simulink model "model"  (R2021a)
settings: Solver=VariableStepAuto  StartTime=0.0  StopTime=100  RelTol=1e-3
values from neighbouring files (symbols this model uses):
  C = eye(12)    [init.m]
  I = [Jx Jxy Jxz ... (first row only)    [init.m]
  m = 1.5    [init.m]
undefined symbols (not defined in the file or in its folder): DiscIntNeverNeededParam, K_lqr, PID_pitch, PID_roll, PID_yaw
libraries: simulink x3
settings Model: Creator=iris  LastModifiedBy=iris

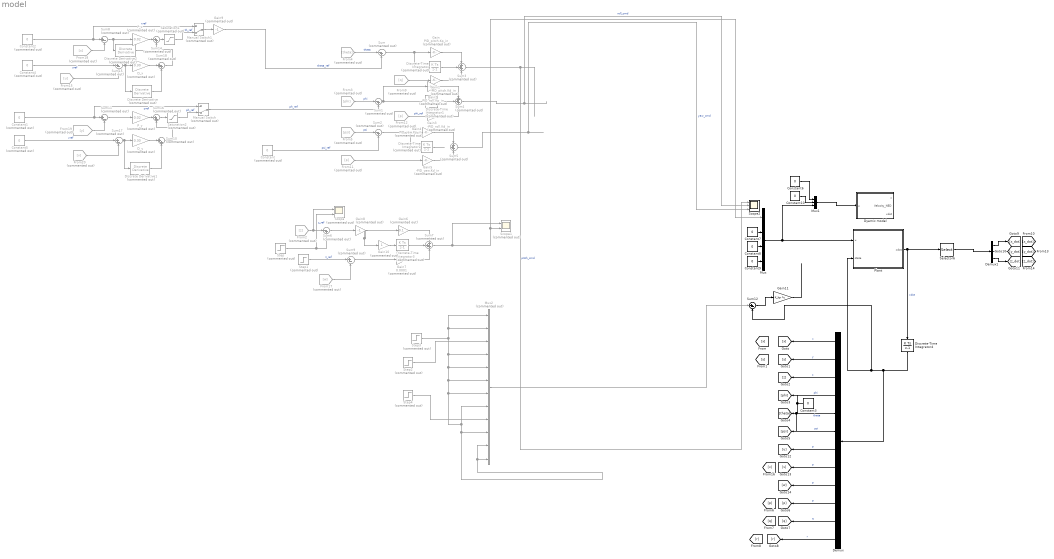
== system model ==
  Constant{,1..2,4..5} (5 alike) : Constant  Commented=on  Value=0
  Constant{3,6..10} (6 alike) : Constant  Value=0
  D_x : Gain  Commented=on  Gain=0.30
  D_y : Gain  Commented=on  Gain=0.30
  Demux : Demux  Outputs=12
  Demux1 : Demux  Outputs=3
  Discrete Derivative : simulink/Discrete/Discrete Derivative  Commented=on  gainval=0.1  ICPrevScaledInput=0.0  OutMin=[]  OutMax=[]  OutDataType=fixdt(1, 16)  OutScaling=2^-10  DoSatur=off
  Discrete Derivative1 : simulink/Discrete/Discrete Derivative  Commented=on  gainval=0.1  ICPrevScaledInput=0.0  OutMin=[]  OutMax=[]  OutDataType=fixdt(1, 16)  OutScaling=2^-10  DoSatur=off
  Discrete Derivative2 : simulink/Discrete/Discrete Derivative  Commented=on  gainval=0.08  ICPrevScaledInput=0.0  OutMin=[]  OutMax=[]  OutDataType=fixdt(1, 16)  OutScaling=2^-10  DoSatur=off
  Discrete-Time Integrator : DiscreteIntegrator  Commented=on  gainval=PID_pitch.Ki_in  SampleTime=-1  ICPrevOutput=DiscIntNeverNeededParam  ICPrevScaledInput=DiscIntNeverNeededParam
  Discrete-Time Integrator1 : DiscreteIntegrator  Commented=on  gainval=PID_roll.Ki_in  SampleTime=-1  ICPrevOutput=DiscIntNeverNeededParam  ICPrevScaledInput=DiscIntNeverNeededParam
  Discrete-Time Integrator2 : DiscreteIntegrator  Commented=on  gainval=PID_yaw.Ki_in  SampleTime=-1  UpperSaturationLimit=0.2  LowerSaturationLimit=-0.2  ICPrevOutput=DiscIntNeverNeededParam  ICPrevScaledInput=DiscIntNeverNeededParam
  Discrete-Time Integrator3 : DiscreteIntegrator  Commented=on  gainval=0.001  SampleTime=-1  ICPrevOutput=DiscIntNeverNeededParam  ICPrevScaledInput=DiscIntNeverNeededParam
  Discrete-Time Integrator4 : DiscreteIntegrator  SampleTime=-1  ICPrevOutput=DiscIntNeverNeededParam  ICPrevScaledInput=DiscIntNeverNeededParam
  Dyamic model : Subsystem
  From11 : From  Commented=on  GotoTag=p
  From12 : From  Commented=on  GotoTag=p
  From15 : From  Commented=on  GotoTag=u
  From17 : From  Commented=on  GotoTag=w
  From18 : From  Commented=on  GotoTag=x
  From19 : From  Commented=on  GotoTag=y
  From2 : From  Commented=on  GotoTag=z
  From20 : From  Commented=on  GotoTag=v
  From3 : From  Commented=on  GotoTag=phi
  From4 : From  Commented=on  GotoTag=theta
  From5 : From  Commented=on  GotoTag=psi
  From9 : From  Commented=on  GotoTag=q
  Gain : Gain  Commented=on  Gain=PID_pitch.Kp_in
  Gain1 : Gain  Commented=on  Gain=-PID_pitch.Kd_in
  Gain10 : Gain  Commented=on
  Gain11 : Gain  Gain=K_lqr  Multiplication=Matrix(K*u)
  Gain2 : Gain  Commented=on  Gain=PID_roll.Kp_in
  Gain3 : Gain  Commented=on  Gain=-PID_roll.Kd_in
  Gain4 : Gain  Commented=on  Gain=PID_yaw.Kp_in
  Gain5 : Gain  Commented=on  Gain=-PID_yaw.Kd_in
  Gain6 : Gain  Commented=on  Gain=0.1
  Gain7 : Gain  Commented=on  Gain=0.0001
  Gain8 : Gain  Commented=on  Gain=-1
  Gain9 : Gain  Commented=on  Gain=-1
  Manual Switch : ManualSwitch  Commented=on  CurrentSetting=0
  Manual Switch1 : ManualSwitch  Commented=on  CurrentSetting=0
  Mux : Mux
  Mux1 : Mux  Inputs=3
  Mux2 : Mux  Commented=on  Inputs=12
  P_x : Gain  Commented=on  Gain=0.02
  P_y : Gain  Commented=on  Gain=0.02
  Plant : Subsystem
  Saturation1 : Saturate  Commented=on  UpperLimit=30/180*pi  LowerLimit=-30/180*pi
  Saturation2 : Saturate  Commented=on  UpperLimit=30/180*pi  LowerLimit=-30/180*pi
  Scope : Scope  Commented=on  NumInputPorts=2
  Scope1 : Scope  Commented=on  NumInputPorts=2
  Scope2 : Scope  NumInputPorts=3
  Selector6 : Selector  InputPortWidth=12  IndexOptions=Index vector (dialog)  Indices=[1:3]  OutputSizes=1
  Step : Step  Commented=on  SampleTime=0
  Step1 : Step  Commented=on  After=0.1  SampleTime=0
  Step2 : Step  Commented=on  SampleTime=0
  Step3 : Step  Commented=on  After=0  SampleTime=0
  Step4 : Step  Commented=on  After=0.1  SampleTime=0
  Sum{,1..2,6} (4 alike) : Sum  Commented=on  Inputs=|-+
  Sum{10,14,16,18} (4 alike) : Sum  Commented=on  Inputs=|++
  Sum{8..9,11,15,17} (5 alike) : Sum  Commented=on  Inputs=|+-
  Sum12 : Sum  Inputs=|+-
  Sum{3..5,7} (4 alike) : Sum  Commented=on  Inputs=+++
  wires:
  Mux/1 -> Plant/1(u), Mux1/3
  Plant/1(xdot) -> Discrete-Time Integrator4/1, Selector6/1  "xdot"
  Demux/1 -> [x]  "x"
  Demux/2 -> [y]  "y"
  Demux/12 -> [r]  "r"
  Demux/4 -> ?  "phi"
  Demux/5 -> ?  "theta"
  Demux/6 -> ?  "psi"
  Demux/10 -> [p]  "p"
  Demux/11 -> [q]  "q"
  From3/1 -> Sum1/1  "phi"
  From5/1 -> Sum2/1  "psi"
  From4/1 -> Sum/1  "theta"
  Demux/3 -> [z]  "z"
  Discrete-Time Integrator/1 -> Sum3/2
  From9/1 -> Gain1/1
  Sum/1 -> Discrete-Time Integrator/1, Gain/1
  Gain1/1 -> Sum3/3
  Constant/1 -> Sum2/2  "psi_ref"
  Gain/1 -> Sum3/1
  Gain3/1 -> Sum4/3
  Gain2/1 -> Sum4/1
  Discrete-Time Integrator1/1 -> Sum4/2
  Sum1/1 -> Gain2/1, Discrete-Time Integrator1/1
  From12/1 -> Gain3/1  "phi_ref"
  Gain4/1 -> Sum5/1
  Sum2/1 -> Discrete-Time Integrator2/1, Gain4/1
  Discrete-Time Integrator2/1 -> ?
  From11/1 -> Gain5/1
  Gain5/1 -> Sum5/3
  Sum3/1 -> Scope2/1  "pitch_cmd"
  Sum4/1 -> Scope2/2  "roll_cmd"
  Sum5/1 -> Scope2/3  "yaw_cmd"
  Discrete-Time Integrator3/1 -> Sum7/2
  Gain6/1 -> Sum7/1
  Gain8/1 -> Gain10/1, Gain6/1
  Gain7/1 -> Sum7/3
  Sum6/1 -> Gain8/1
  Selector6/1 -> Demux1/1
  Demux1/1 -> [x_dot]
  Demux1/2 -> [y_dot]
  Demux1/3 -> [z_dot]
  From17/1 -> Sum9/2
  From2/1 -> Scope/1, Sum6/1
  Step/1 -> Scope/2, Sum6/2  "z_ref"
  Gain9/1 -> Sum/2  "theta_ref"
  Demux/7 -> [u]  "p"
  Demux/8 -> [v]  "p"
  Demux/9 -> [w]  "p"
  Manual Switch1/1 -> Gain9/1
  Sum17/1 -> Discrete Derivative1/1, D_y/1
  From18/1 -> Sum8/2
  Saturation2/1 -> Manual Switch/2  "ph_ref"
  Constant4/1 -> Sum15/1  "uref"
  Constant5/1 -> Sum17/1  "vref"
  From20/1 -> Sum17/2
  Sum10/1 -> Sum16/2
  Discrete Derivative/1 -> Sum18/2
  Sum11/1 -> P_y/1
  Discrete Derivative2/1 -> ?
  Sum8/1 -> Discrete Derivative2/1, P_x/1
  P_x/1 -> Sum14/1
  D_y/1 -> Sum10/1
  Discrete Derivative1/1 -> Sum10/2
  Saturation1/1 -> Manual Switch1/2  "th_ref"
  Sum15/1 -> Discrete Derivative/1, D_x/1
  From15/1 -> Sum15/2
  Constant2/1 -> Manual Switch1/1, Sum8/1  "xref"
  Constant1/1 -> Manual Switch/1, Sum11/1  "yref"
  From19/1 -> Sum11/2
  D_x/1 -> Sum18/1
  Sum14/1 -> Saturation1/1
  Manual Switch/1 -> Sum1/2  "ph_ref"
  P_y/1 -> Sum16/1
  Sum16/1 -> Saturation2/1
  Sum18/1 -> Sum14/2
  Constant7/1 -> Mux/2
  Constant8/1 -> Mux/3
  Constant9/1 -> Mux/4
  Sum9/1 -> Gain7/1
  Sum7/1 -> Mux/1, Scope1/2, Scope1/1
  Step1/1 -> Sum9/1  "z_ref"
  Constant3/1 -> [psi], [theta], [phi]
  Constant10/1 -> Mux1/2
  Constant6/1 -> Mux1/1
  Mux1/1 -> Dyamic model/1(u)
  Gain10/1 -> Discrete-Time Integrator3/1
  Mux2/1 -> Sum12/1
  Sum12/1 -> Gain11/1
  Discrete-Time Integrator4/1 -> Demux/1, Sum12/2, Plant/2(state)
  Gain11/1 -> ?
  Step3/1 -> Mux2/2, Mux2/1, Mux2/11, Mux2/12, Mux2/10, Mux2/8, Mux2/7, Mux2/6, Mux2/5, Mux2/4
  Step2/1 -> Mux2/3
  Step4/1 -> Mux2/9

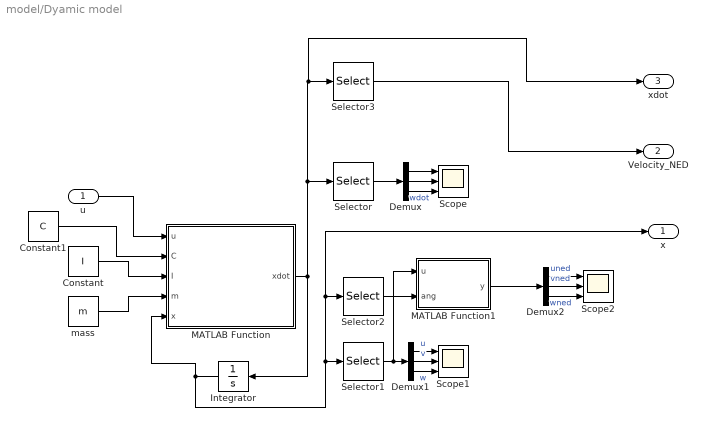
== system model/Dyamic model ==
  u : Inport
  Constant : Constant  Value=I
  Constant1 : Constant  Value=C
  Demux : Demux  Outputs=3
  Demux1 : Demux  Outputs=3
  Demux2 : Demux  Outputs=3
  Integrator : Integrator
  MATLAB Function : MATLAB Function  TreatAsAtomicUnit=on
  MATLAB Function1 : MATLAB Function  TreatAsAtomicUnit=on
  Scope : Scope  NumInputPorts=3
  Scope1 : Scope  NumInputPorts=3
  Scope2 : Scope  NumInputPorts=3
  Selector : Selector  InputPortWidth=12  IndexOptions=Index vector (dialog)  Indices=[7:9]  OutputSizes=1
  Selector1 : Selector  InputPortWidth=12  IndexOptions=Index vector (dialog)  Indices=[7:9]  OutputSizes=1
  Selector2 : Selector  InputPortWidth=12  IndexOptions=Index vector (dialog)  Indices=[4:6]  OutputSizes=1
  Selector3 : Selector  InputPortWidth=12  IndexOptions=Index vector (dialog)  Indices=[1:3]  OutputSizes=1
  mass : Constant  Value=m
  x : Outport  VectorParamsAs1DForOutWhenUnconnected=off
  Velocity_NED : Outport  Port=2  VectorParamsAs1DForOutWhenUnconnected=off
  xdot : Outport  Port=3  VectorParamsAs1DForOutWhenUnconnected=off
  wires:
  mass/1 -> MATLAB Function/4(m)
  MATLAB Function/1(xdot) -> xdot/1, Selector3/1, Selector/1, Integrator/1
  u/1 -> MATLAB Function/1(u)
  Constant/1 -> MATLAB Function/3(I)
  Demux/1 -> Scope/1
  Demux/2 -> Scope/2
  Demux/3 -> Scope/3  "wdot"
  Selector/1 -> Demux/1
  Integrator/1 -> Selector2/1, x/1, Selector1/1, MATLAB Function/5(x)
  Selector1/1 -> MATLAB Function1/1(u), Demux1/1
  Demux1/1 -> Scope1/1  "u"
  Demux1/2 -> Scope1/2  "v"
  Demux1/3 -> Scope1/3  "w"
  Demux2/1 -> Scope2/1  "uned"
  Demux2/2 -> Scope2/2  "vned"
  Demux2/3 -> Scope2/3  "wned"
  MATLAB Function1/1(y) -> Demux2/1
  Selector2/1 -> MATLAB Function1/2(ang)
  Selector3/1 -> Velocity_NED/1
  Constant1/1 -> MATLAB Function/2(C)

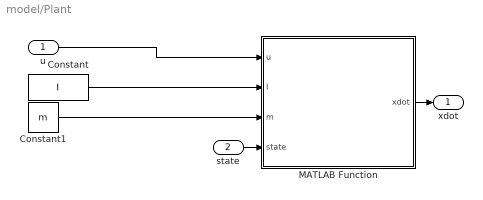
== system model/Plant ==
  u : Inport
  state : Inport  Port=2
  Constant : Constant  Value=I
  Constant1 : Constant  Value=m
  MATLAB Function : MATLAB Function  TreatAsAtomicUnit=on
  xdot : Outport
  wires:
  u/1 -> MATLAB Function/1(u)
  Constant1/1 -> MATLAB Function/3(m)
  MATLAB Function/1(xdot) -> xdot/1
  Constant/1 -> MATLAB Function/2(I)
  state/1 -> MATLAB Function/4(state)

== matlab function model/Dyamic model/MATLAB Function ==
  data: u input; C input; I input; m input; x input; xdot output
function xdot = quadrotor_dynamics(u,C,I,m,x)

ph = x(4);
th = x(5);
ps = x(6);
U = x(7);
V = x(8);
W = x(9);
p = x(10);
q = x(11);
r = x(12);
% Rotation from body to NED
% Rb_ned = [cos(th)*cos(ps), -cos(ph)*sin(ps) + sin(ph)*sin(th)*...
%                 cos(ps), sin(ph)*sin(ps) + cos(ph)*sin(th)*cos(ps)
%             cos(th)*sin(ps), cos(ph)*sin(th)*cos(ps), -sin(ph)*...
%                 cos(ps) + cos(ph)*sin(th)*sin(ps)
%             sin(th), -sin(ph)*cos(th), -cos(ph)*cos(th) ];
        
% Rb_ned = [ cos(ph)*cos(ps), cos(th)*sin(ph), -sin(th)
%             cos(ps)*sin(th)*sin(ps) - cos(ps)*sin(ph), cos(ps)*...
%                 cos(ph) + sin(ph)*sin(th)*sin(ps), cos(th)*sin(ps)
%             sin(ph)*sin(ps) + cos(ph)*cos(ps)*sin(th), cos(ps)*...
%                 sin(ph)*sin(th) - cos(ph)*sin(ps), cos(th)*cos(ps) ];
            
Rb_ned = [ cos(th)*cos(ps), cos(th)*sin(ps), -sin(th)
            -cos(ph)*sin(ps) + sin(ph)*sin(th)*cos(ps), cos(ph)...
                *cos(ps) + sin(ph)*sin(th)*sin(ps), sin(ph)*cos(th)
            sin(ph)*sin(ps) + cos(ph)*sin(th)*cos(ps), -sin(ph)...
            *cos(ps) + cos(ph)*sin(th)*sin(ps), cos(ph)*cos(th) ];
% Rb_ned = zeros(3,3);        
% Rb_ned(1,:) = [cos(ps)*cos(th) -sin(th)*cos(ph)+cos(ps)*sin(th)*sin(ph) sin(ps)*sin(ph)+cos(ps)*cos(ph)*sin(th)];
% Rb_ned(2,:) = [sin(ps)*cos(th) cos(ps)*cos(ph)+sin(ps)*sin(th)*sin(ps) -cos(ps)*sin(ph)+sin(th)*sin(ps)*cos(ph)];
% Rb_ned(3,:) = [-sin(th) cos(th)*sin(ph) cos(th)*cos(ph)];
% Constants linked to Inertia Moments
c1 = C(1);
c2 = C(2);
c3 = C(3);
c4 = C(4);
c5 = C(5);
c6 = C(6);
c7 = C(7);
c8 = C(8);
c9 = C(9);
% Non-linear plant in the form x_dot = f(x) + g(x)*u
f = [ Rb_ned'*x(7:9)
        p + tan(th)*(q*sin(ph) + r*cos(ph))
        q*cos(ph) - r*sin(ph)
        1/cos(th)*(q*sin(ph) + r*cos(ph))
        r*V - q*W - 9.81*sin(th)
        -r*U + p*W + 9.81*sin(ph)*cos(th)
        q*U - p*V + 9.81*cos(ph)*cos(th)
        (c1*r + c2*p)*q
        c5*p*r - c6*(p^2 - r^2) 
        (c8*p - c2*r)*q ];

g = zeros(12,6);
g(7:9,1:3) = diag([1/m,1/m,1/m]);
g(10,4) = c3;
g(10,6) = c4;
g(11,5) = c7;
g(12,4) = c4;
g(12,6) = c9;
% i_1 = (I(2,2)-I(3,3))/I(1,1);
% i_2 = 1/I(1,1);
% i_3 = (I(3,3)-I(1,1))/I(2,2);
% i_4 = 1/I(2,2);
% i_5 = (I(1,1)-I(2,2))/I(3,3);
% i_6 = 1/I(3,3);
% 
% g = zeros(12,4);
% g(10,2) = i_2;
% g(11,3) = i_4;
% g(12,4) = i_6;

xdot = f + g*u;
end

== matlab function model/Plant/MATLAB Function ==
  data: u input; xdot output; I input; m input; state input
function xdot = plant(u,I,m,state)

grav = 9.81;
T = u(1);
U = state(7);
V = state(8);
W = state(9);
phi = state(4);
th  = state(5);
psi = state(6);
p  = state(10);
q  = state(11);
r  = state(12);

i_1 = (I(2,2)-I(3,3))/I(1,1);
i_2 = 1/I(1,1);
i_3 = (I(3,3)-I(1,1))/I(2,2);
i_4 = 1/I(2,2);
i_5 = (I(1,1)-I(2,2))/I(3,3);
i_6 = 1/I(3,3);


Rot_mat = [cos(th)*cos(psi) sin(phi)*sin(th)*cos(psi)-cos(phi)*sin(psi) cos(phi)*sin(th)*cos(psi)+sin(phi)*sin(psi);
    cos(th)*sin(psi) sin(phi)*sin(th)*sin(psi)+cos(phi)*cos(psi) cos(phi)*sin(th)*sin(psi)-sin(phi)*cos(psi);
    -sin(th) sin(phi)*cos(th) cos(phi)*cos(th)]; % body to NED


f = [Rot_mat*state(7:9)
     p + (sin(phi)*tan(th))*q - (cos(phi)*tan(th))*r
     cos(phi)*q + sin(phi)*r
     -1*sin(phi)*sec(th)*q + cos(phi)*sec(th)*r
     0
     0
%      r*V - q*W - 9.81*sin(th)
%      -r*U + p*W + 9.81*sin(phi)*cos(th)
%      q*U - p*V + 9.81*cos(phi)*cos(th)
%      -1/m*(cos(phi)*sin(th)*cos(psi) + sin(phi)*sin(psi))%*T
%      -1/m*(cos(phi)*sin(th)*sin(psi) - sin(phi)*cos(psi))%*T
     grav - 1/m*(cos(phi)*cos(th))*T
     i_1*q*r
     i_3*r*p
     i_5*p*q];
        

g = zeros(12,4);
% g(7,1) = -1/m*(cos(phi)*sin(th)*cos(psi) + sin(phi)*sin(psi));
% g(8,1) = -1/m*(cos(phi)*sin(th)*sin(psi) - sin(phi)*cos(psi));
% g(9,1) = - 1/m*(cos(phi)*cos(th));
g(10,2) = i_2;
g(11,3) = i_4;
g(12,4) = i_6;

xdot = f + g*u;

end

== matlab function model/Dyamic model/MATLAB Function1 ==
  data: u input; y output; ang input
function y = fcn(u,ang)

ph = ang(1);
th = ang(2);
ps = ang(3);

Rb_ned = [ cos(th)*cos(ps), cos(th)*sin(ps), -sin(th)
            -cos(ph)*sin(ps) + sin(ph)*sin(th)*cos(ps), cos(ph)...
                *cos(ps) + sin(ph)*sin(th)*sin(ps), sin(ph)*cos(th)
            sin(ph)*sin(ps) + cos(ph)*sin(th)*cos(ps), -sin(ph)...
            *cos(ps) + cos(ph)*sin(th)*sin(ps), cos(ph)*cos(th) ];
        
y = Rb_ned'*u;

end
